simulink model "blank01"  (Simulink 7.4)
settings: Solver=ode45  StartTime=0.0  StopTime=inf  RelTol=1e-3
libraries: NAV420Lib x1
settings Model: Creator=djulzz  LastModifiedBy=djulzz

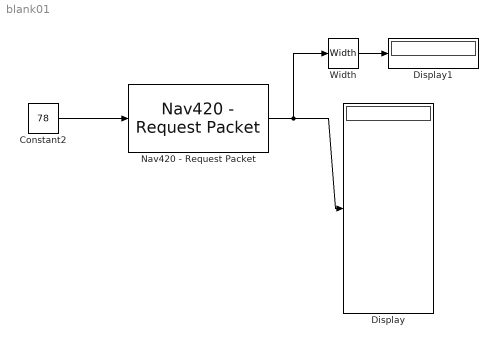
== system blank01 ==
  Constant2 : Constant  Value=78  OutDataTypeMode=int8  OutDataType=fixdt(1, 16)  OutScaling=2^0  OutDataTypeStr=int8  SampleTime=-1
  Display : Display
      settings: Format=hex (Stored Integer)
  Display1 : Display
  Nav420 - Request Packet : NAV420Lib/Nav420 - Request Packet  SystemSampleTime=-1
  Width : Width
  wires:
  Constant2/1 -> Nav420 - Request Packet/1
  Nav420 - Request Packet/1 -> Display/1, Width/1
  Width/1 -> Display1/1
